simulink model "comp_model"  (R2021a)
settings: Solver=ode3  StartTime=0.0  StopTime=1  FixedStep=0.01  RelTol=1e-3
values from neighbouring files (symbols this model uses):
  A = [0 1 0 0; -K_m/M 0 K_m/M 0; 0 0 0 1; K_m/M 0 -K_m/M 0]    [desafio1.m]
  B = [0 0; 1/M 0; 0 0; 0 1/M]    [desafio1.m]
  C = [1 0 0 0; 0 0 1 0]    [desafio1.m]
  F = -place(A , B, pF)    [desafio1.m]
  K = place(A.',C.',pK*120)'    [desafio1.m]
  r = [1; 5]    [desafio1.m]
  sim_step = 0.01    [desafio1.m]
  x0 = [0; 0; 0; 0]    [desafio1.m]
libraries: simulink x1
settings Model: Creator=Murillo  LastModifiedBy=vinic
settings SolverCC: AlgebraicLoopSolver=TrustRegion
settings OptimizationCC: LifeSpan=inf
settings DebuggingCC: SFExecutionAtInitializationDiag=none  SFMachineParentedDataDiag=warning  ArithmeticOperatorsInVariantConditions=warning
settings HardwareCC: ProdBitPerSizeT=32  ProdBitPerPtrDiffT=32  ProdWordSize=32  ProdHWDeviceType=Specified
settings SFSimCC: CustomCodeUndefinedFunction=UseInterfaceOnly
settings CodeAppCC: StateflowObjectComments=on

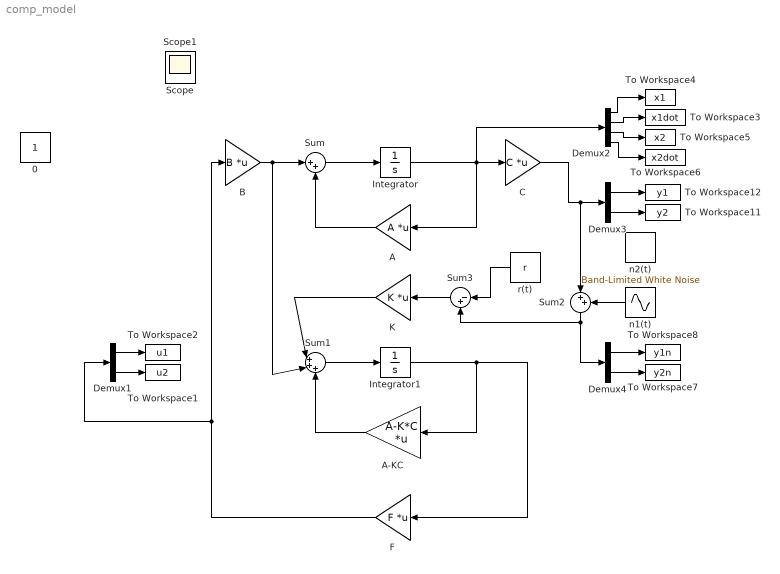
== system comp_model ==
  A : Gain  Gain=A  Multiplication=Matrix(K*u)
  A-KC : Gain  Gain=A-K*C  Multiplication=Matrix(K*u)
  B : Gain  Gain=B  Multiplication=Matrix(K*u)
  C : Gain  Gain=C  Multiplication=Matrix(K*u)
  Demux1 : Demux  Outputs=2
  Demux2 : Demux
  Demux3 : Demux  Outputs=2
  Demux4 : Demux  Outputs=2
  F : Gain  Gain=F  Multiplication=Matrix(K*u)
  Integrator : Integrator  InitialCondition=x0
  Integrator1 : Integrator
  K : Gain  Gain=K  Multiplication=Matrix(K*u)
  Sum : Sum  Inputs=|++
  Sum1 : Sum  Inputs=|+++
  Sum2 : Sum  Inputs=|++
  Sum3 : Sum  Inputs=|-+
  To Workspace1 : ToWorkspace  VariableName=u2  SampleTime=-1
      settings: Save2DSignal=2-D array (concatenate along first dimension)
  To Workspace11 : ToWorkspace  VariableName=y2  SampleTime=-1
      settings: Save2DSignal=2-D array (concatenate along first dimension)
  To Workspace12 : ToWorkspace  VariableName=y1  SampleTime=-1
      settings: Save2DSignal=2-D array (concatenate along first dimension)
  To Workspace2 : ToWorkspace  VariableName=u1  SampleTime=-1
      settings: Save2DSignal=2-D array (concatenate along first dimension)
  To Workspace3 : ToWorkspace  VariableName=x1dot  SampleTime=-1
      settings: Save2DSignal=2-D array (concatenate along first dimension)
  To Workspace4 : ToWorkspace  VariableName=x1  SampleTime=-1
      settings: Save2DSignal=2-D array (concatenate along first dimension)
  To Workspace5 : ToWorkspace  VariableName=x2  SampleTime=-1
      settings: Save2DSignal=2-D array (concatenate along first dimension)
  To Workspace6 : ToWorkspace  VariableName=x2dot  SampleTime=-1
      settings: Save2DSignal=2-D array (concatenate along first dimension)
  To Workspace7 : ToWorkspace  VariableName=y2n  SampleTime=-1
      settings: Save2DSignal=2-D array (concatenate along first dimension)
  To Workspace8 : ToWorkspace  VariableName=y1n  SampleTime=-1
      settings: Save2DSignal=2-D array (concatenate along first dimension)
  n1(t) : Sin  Amplitude=0.01  Frequency=100  SampleTime=0
  n2(t) : simulink/Sources/Band-Limited White Noise  Cov=[1e-4]  Ts=sim_step  seed=[23341]
  r(t) : Constant  Value=r  VectorParams1D=off
  0 : Constant  IOType=siggen
  Scope : Scope
  Scope1 : Scope
  wires:
  Sum/1 -> Integrator/1
  A/1 -> Sum/2
  B/1 -> Sum/1, Sum1/2
  Sum1/1 -> Integrator1/1
  Integrator1/1 -> A-KC/1, F/1
  A-KC/1 -> Sum1/3
  F/1 -> B/1, Demux1/1
  K/1 -> Sum1/1
  r(t)/1 -> Sum3/1
  Integrator/1 -> A/1, Demux2/1, C/1
  Demux2/2 -> To Workspace3/1
  Demux2/4 -> To Workspace6/1
  Demux2/1 -> To Workspace4/1
  Demux2/3 -> To Workspace5/1
  Demux1/1 -> To Workspace2/1
  Demux1/2 -> To Workspace1/1
  C/1 -> Demux3/1, Sum2/1
  Demux3/2 -> To Workspace11/1
  Demux3/1 -> To Workspace12/1
  Demux4/2 -> To Workspace7/1
  Demux4/1 -> To Workspace8/1
  Sum2/1 -> Demux4/1, Sum3/2
  Sum3/1 -> K/1
  n1(t)/1 -> Sum2/2
